simulink model "SatelliteServicing_Mission_RigidBodyTree"  (R2022a)
settings: Solver=ode15s  StartTime=0.0  StopTime=endTime  RelTol=1e-3
libraries: nesl_utility x18, sm_lib x3, robotmaniplib x2
settings Model: Creator=Andy  LastModifiedBy=Andy
settings DebuggingCC: UnconnectedInputMsg=warning  UnconnectedOutputMsg=warning  UnconnectedLineMsg=warning
settings RTWCC: DLArmComputeVersion=19.05
settings SimscapeCC: SimscapeLogType=all

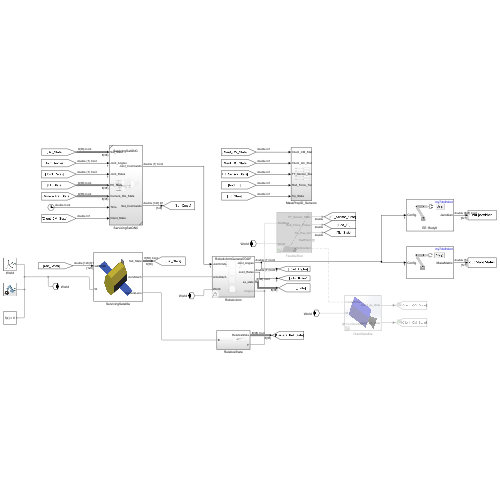
[thumbnail: Simulink's stored preview of the top-level diagram]
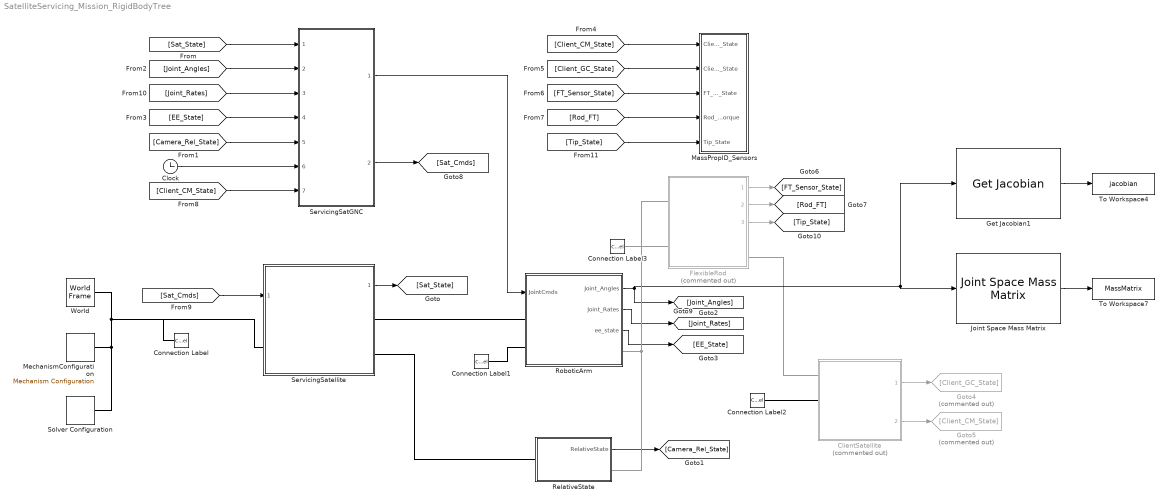
== system SatelliteServicing_Mission_RigidBodyTree ==
  ClientSatellite : Subsystem  Commented=on  ReferencedSubsystem=ClientSatellite
  Clock : Clock
  Connection Label{,1..3} (4 alike) : ConnectionLabel  Label=World
  FlexibleRod : Subsystem  Commented=on  ReferencedSubsystem=FlexibleRodModel
  Get Jacobian1 : robotmaniplib/Get Jacobian  RigidBodyTree=my7dofrobot  EndEffector=Body8  SimulateUsing=Interpreted execution
      settings: SourceProductBaseCode=RO
  Goto4 : Goto  Commented=on  GotoTag=Client_GC_State
  Goto5 : Goto  Commented=on  GotoTag=Client_CM_State
  Joint Space Mass Matrix : robotmaniplib/Joint Space Mass Matrix  RigidBodyTree=my7dofrobot  SimulateUsing=Interpreted execution
  MassPropID_Sensors : Subsystem
  MechanismConfiguration : sm_lib/Utilities/Mechanism Configuration  UniformGravity=Constant  GravityVector=[0 0 -9.80665]*0  GravityUnits=m/s^2  LinearizationDelta=0.001  JointModeTransitionNonlinearIterations=2
  RelativeState : Subsystem
  RoboticArm : Subsystem  Variant=on  VariantControl=Choice
  ServicingSatGNC : Subsystem  SystemSampleTime=0.001  ReferencedSubsystem=ServicingSatGNC
      settings: MinAlgLoopOccurrences=on
  ServicingSatellite : Subsystem  ReferencedSubsystem=ServicingSatellite
  Solver Configuration : nesl_utility/Solver Configuration  PhysicalDomain=network_engine_domain  SubClassName=solver  LeftPortType=input  RightPortType=generic  Tones=[]  Harmonics=[]  SimulateNoise=off  Profile=off  UseLocalSampling=off  EnableSwitchedLinearOptims=on  FrequencyDomain=off  UseCCode=off  RelTol=0.001  AbsTol=1e-06  MinStep=1e-09  ToWorkspace=off  RevertToSquareIcSolve=off  NumHomotopyIterations=100  PhasorMode=off  PhasorModeNumHarmonics=1  IndexReductionMethod=DerivativeReplacement  DoDC=off  ResidualTolerance=1e-09  UseLocalSolver=off  LocalSolverChoice=NE_BACKWARD_EULER_ADVANCER  LocalSolverSampleTime=0.001  DoFixedCost=off  MaxNonlinIter=3  MaxModeIter=2  ComputeImpulses=off  ImpulseIterations=2  LinearAlgebra=auto  LinearAlgebraNumThread=0  EquationFormulation=NE_TIME_EF  DelaysMemoryBudget=1024  AutomaticFiltering=on  FilteringTimeConstant=0.001  PartitionStorageMethod=AS_NEEDED  PartitionMemoryBudget=1024  PartitionMethod=ROBUST
      settings: SourceProductBaseCode=SS,PW,VE
  To Workspace4 : ToWorkspace  VariableName=jacobian  SaveFormat=Timeseries  SampleTime=-1
  To Workspace7 : ToWorkspace  VariableName=MassMatrix  SaveFormat=Timeseries  SampleTime=-1
  World : sm_lib/Frames and Transforms/World Frame
  wires:
  ServicingSatellite/1 -> [Sat_State]
  RelativeState/1(RelativeState) -> [Camera_Rel_State]
  ClientSatellite/1 -> Goto4/1
  FlexibleRod/1 -> [FT_Sensor_State]
  FlexibleRod/2 -> [Rod_FT]
  [Client_CM_State] -> MassPropID_Sensors/1(Client_CM_State)
  [Client_GC_State] -> MassPropID_Sensors/2(Client_GC_State)
  [FT_Sensor_State] -> MassPropID_Sensors/3(FT_Sensor_State)
  [Rod_FT] -> MassPropID_Sensors/4(Rod_Force_Torque)
  [Sat_Cmds] -> ServicingSatellite/1
  ServicingSatGNC/2 -> [Sat_Cmds]
  [Client_CM_State] -> ServicingSatGNC/7
  [Camera_Rel_State] -> ServicingSatGNC/5
  [EE_State] -> ServicingSatGNC/4
  [Sat_State] -> ServicingSatGNC/1
  [Joint_Angles] -> ServicingSatGNC/2
  Clock/1 -> ServicingSatGNC/6
  [Joint_Rates] -> ServicingSatGNC/3
  ServicingSatGNC/1 -> RoboticArm/1(JointCmds)
  RoboticArm/1(Joint_Angles) -> [Joint_Angles], Get Jacobian1/1, Joint Space Mass Matrix/1
  RoboticArm/2(Joint_Rates) -> [Joint_Rates]
  RoboticArm/3(ee_state) -> [EE_State]
  FlexibleRod/3 -> [Tip_State]
  [Tip_State] -> MassPropID_Sensors/5(Tip_State)
  ClientSatellite/2 -> Goto5/1
  Get Jacobian1/1 -> To Workspace4/1
  Joint Space Mass Matrix/1 -> To Workspace7/1
  connections:
  MechanismConfiguration/RConn1 -- ServicingSatellite/LConn1 -- Connection Label/LConn1 -- World/RConn1 -- Solver Configuration/RConn1
  FlexibleRod/RConn2 -- ClientSatellite/LConn1
  RelativeState/LConn1 -- ServicingSatellite/RConn2
  Connection Label2/LConn1 -- ClientSatellite/LConn2
  FlexibleRod/LConn2 -- Connection Label3/LConn1
  RoboticArm/LConn1 -- ServicingSatellite/RConn1
  RoboticArm/LConn2 -- Connection Label1/LConn1
  FlexibleRod/LConn1 -- RelativeState/RConn1 -- RoboticArm/RConn1

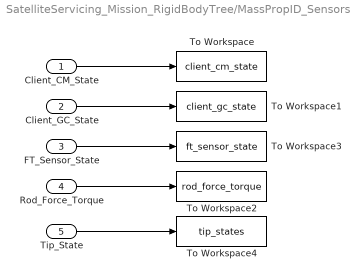
== system SatelliteServicing_Mission_RigidBodyTree/MassPropID_Sensors ==
  Client_CM_State : Inport
  Client_GC_State : Inport  Port=2
  FT_Sensor_State : Inport  Port=3
  Rod_Force_Torque : Inport  Port=4
  Tip_State : Inport  Port=5
  To Workspace : ToWorkspace  VariableName=client_cm_state  SaveFormat=Timeseries  SampleTime=-1
  To Workspace1 : ToWorkspace  VariableName=client_gc_state  SaveFormat=Timeseries  SampleTime=-1
  To Workspace2 : ToWorkspace  VariableName=rod_force_torque  SaveFormat=Timeseries  SampleTime=-1
  To Workspace3 : ToWorkspace  VariableName=ft_sensor_state  SaveFormat=Timeseries  SampleTime=-1
  To Workspace4 : ToWorkspace  VariableName=tip_states  SaveFormat=Timeseries  SampleTime=-1
  wires:
  Rod_Force_Torque/1 -> To Workspace2/1
  Client_CM_State/1 -> To Workspace/1
  Client_GC_State/1 -> To Workspace1/1
  FT_Sensor_State/1 -> To Workspace3/1
  Tip_State/1 -> To Workspace4/1

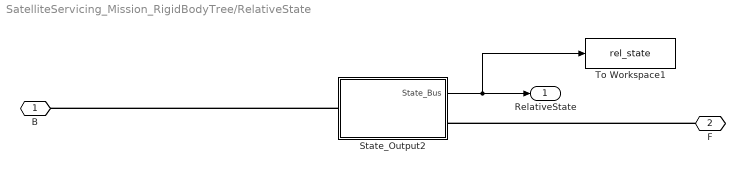
== system SatelliteServicing_Mission_RigidBodyTree/RelativeState ==
  State_Output2 : Subsystem
  To Workspace1 : ToWorkspace  VariableName=rel_state  SaveFormat=Timeseries  SampleTime=-1
  B : PMIOPort  Side=Left
  F : PMIOPort  Port=2  Side=Right
  RelativeState : Outport
  wires:
  State_Output2/1(State_Bus) -> To Workspace1/1, RelativeState/1
  connections:
  F/RConn1 -- State_Output2/RConn1
  State_Output2/LConn1 -- B/RConn1

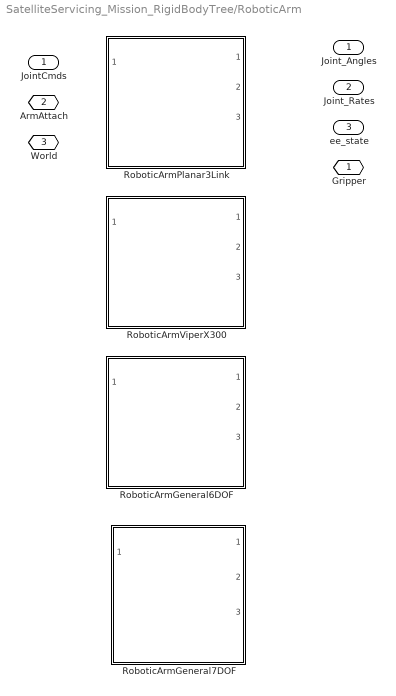
== system SatelliteServicing_Mission_RigidBodyTree/RoboticArm ==
  JointCmds : Inport
  RoboticArmGeneral6DOF : Subsystem  VariantControl=VSS_RoboticArmGeneral6DOF  ReferencedSubsystem=RoboticArmGeneral6DOF
  RoboticArmGeneral7DOF : Subsystem  VariantControl=VSS_RoboticArmGeneral7DOF  ReferencedSubsystem=RoboticArmGeneral7DOF
  RoboticArmPlanar3Link : Subsystem  VariantControl=VSS_RoboticArmPlanar3Link  ReferencedSubsystem=RoboticArmPlanar3Link
  RoboticArmViperX300 : Subsystem  VariantControl=VSS_RoboticArmViperX300  ReferencedSubsystem=RoboticArmViperX300
  Gripper : PMIOPort  Side=Right
  ArmAttach : PMIOPort  Port=2  Side=Left
  World : PMIOPort  Port=3  Side=Left
  Joint_Angles : Outport
  Joint_Rates : Outport  Port=2
  ee_state : Outport  Port=3

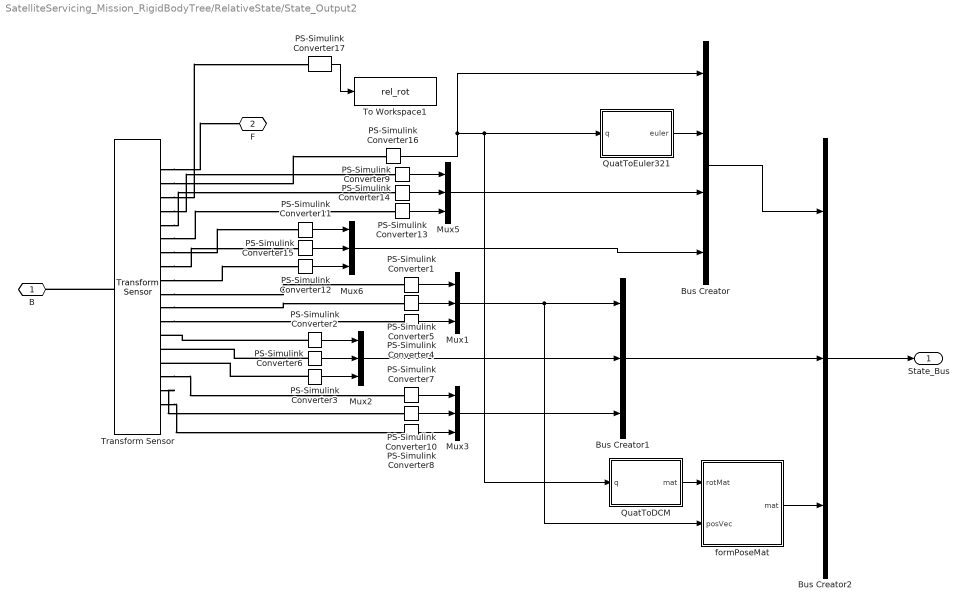
== system SatelliteServicing_Mission_RigidBodyTree/RelativeState/State_Output2 ==
  Bus Creator : BusCreator  Inputs=4  OutDataTypeStr=Bus: RotStateBus
      settings: InheritFromInputs=off
  Bus Creator1 : BusCreator  Inputs=3  OutDataTypeStr=Bus: TransStateBus
      settings: InheritFromInputs=off
  Bus Creator2 : BusCreator  Inputs=3  OutDataTypeStr=Bus: StateBus
      settings: InheritFromInputs=off
  Mux{1..3,5..6} (5 alike) : Mux  Inputs=3
  PS-Simulink Converter{1..17} (17 alike) : nesl_utility/PS-Simulink Converter  PhysicalDomain=network_engine_domain  SubClassName=ps_output  LeftPortType=input  RightPortType=output  PseudoPeriodic=off  Frequencies=[]  VectorFormat=1-D array  Unit=inherit  AffineConversion=off
      settings: SourceProductBaseCode=SS,PW,VE
  QuatToDCM : MATLAB Function  TreatAsAtomicUnit=on
  QuatToEuler321 : MATLAB Function  TreatAsAtomicUnit=on
  To Workspace1 : ToWorkspace  VariableName=rel_rot  SaveFormat=Timeseries  SampleTime=-1
  Transform Sensor : sm_lib/Frames and Transforms/Transform Sensor  MeasurementFrame=Base  SenseAngle=off  SenseAxis=off  SenseAngle1=off  SenseAngle2=off  SenseAngle3=off  SenseQ=on  SenseR=on  SenseOmegaX=on  SenseOmegaY=on  SenseOmegaZ=on  SenseOmega1=off  SenseOmega2=off  SenseOmega3=off  SenseQDot=off  SenseRDot=off  SenseAlphaX=on  SenseAlphaY=on  SenseAlphaZ=on  SenseAlpha1=off  SenseAlpha2=off  SenseAlpha3=off  SenseQDDot=off  SenseRDDot=off  SenseX=on  SenseY=on  SenseZ=on  SenseRad=off  SenseAzim=off  SenseDist=off  SenseInc=off  SenseXDot=on  SenseYDot=on  SenseZDot=on  SenseRadDot=off  SenseAzimDot=off  SenseDistDot=off  SenseIncDot=off  SenseXDDot=on  SenseYDDot=on  SenseZDDot=on  SenseRadDDot=off  SenseAzimDDot=off  SenseDistDDot=off  SenseIncDDot=off
  formPoseMat : MATLAB Function  TreatAsAtomicUnit=on
  B : PMIOPort  Side=Left
  F : PMIOPort  Port=2  Side=Right
  State_Bus : Outport
  wires:
  PS-Simulink Converter4/1 -> Mux1/3
  PS-Simulink Converter5/1 -> Mux1/2
  PS-Simulink Converter1/1 -> Mux1/1
  PS-Simulink Converter3/1 -> Mux2/3
  PS-Simulink Converter6/1 -> Mux2/2
  PS-Simulink Converter2/1 -> Mux2/1
  PS-Simulink Converter10/1 -> Mux3/2
  PS-Simulink Converter8/1 -> Mux3/3
  PS-Simulink Converter7/1 -> Mux3/1
  Mux2/1 -> Bus Creator1/2
  Mux1/1 -> formPoseMat/2(posVec), Bus Creator1/1
  Mux3/1 -> Bus Creator1/3
  PS-Simulink Converter9/1 -> Mux5/1
  PS-Simulink Converter14/1 -> Mux5/2
  PS-Simulink Converter13/1 -> Mux5/3
  Mux5/1 -> Bus Creator/3
  PS-Simulink Converter15/1 -> Mux6/2
  PS-Simulink Converter12/1 -> Mux6/3
  Mux6/1 -> Bus Creator/4
  PS-Simulink Converter11/1 -> Mux6/1
  PS-Simulink Converter16/1 -> QuatToEuler321/1(q), QuatToDCM/1(q), Bus Creator/1
  QuatToEuler321/1(euler) -> Bus Creator/2
  Bus Creator/1 -> Bus Creator2/1
  Bus Creator1/1 -> Bus Creator2/2
  Bus Creator2/1 -> State_Bus/1
  QuatToDCM/1(mat) -> formPoseMat/1(rotMat)
  formPoseMat/1(mat) -> Bus Creator2/3
  PS-Simulink Converter17/1 -> To Workspace1/1
  connections:
  Transform Sensor/LConn1 -- B/RConn1
  Transform Sensor/RConn1 -- F/RConn1
  Transform Sensor/RConn10 -- PS-Simulink Converter1/LConn1
  Transform Sensor/RConn11 -- PS-Simulink Converter5/LConn1
  Transform Sensor/RConn12 -- PS-Simulink Converter4/LConn1
  PS-Simulink Converter3/LConn1 -- Transform Sensor/RConn15
  PS-Simulink Converter6/LConn1 -- Transform Sensor/RConn14
  PS-Simulink Converter2/LConn1 -- Transform Sensor/RConn13
  Transform Sensor/RConn18 -- PS-Simulink Converter8/LConn1
  Transform Sensor/RConn16 -- PS-Simulink Converter7/LConn1
  Transform Sensor/RConn17 -- PS-Simulink Converter10/LConn1
  Transform Sensor/RConn9 -- PS-Simulink Converter12/LConn1
  Transform Sensor/RConn6 -- PS-Simulink Converter13/LConn1
  Transform Sensor/RConn5 -- PS-Simulink Converter14/LConn1
  Transform Sensor/RConn4 -- PS-Simulink Converter9/LConn1
  Transform Sensor/RConn8 -- PS-Simulink Converter15/LConn1
  Transform Sensor/RConn7 -- PS-Simulink Converter11/LConn1
  Transform Sensor/RConn2 -- PS-Simulink Converter16/LConn1
  Transform Sensor/RConn3 -- PS-Simulink Converter17/LConn1

== matlab function SatelliteServicing_Mission_RigidBodyTree/RelativeState/State_Output2/QuatToDCM ==
  data: q input; mat output
function mat  = callQuatToDCM(q)

[mat] = simscapeQuatToDCM(q);

== matlab function SatelliteServicing_Mission_RigidBodyTree/RelativeState/State_Output2/QuatToEuler321 ==
  data: q input; euler output
function euler  = callQuatToEuler321(q)


[euler] = quatToEuler_321(q);

== matlab function SatelliteServicing_Mission_RigidBodyTree/RelativeState/State_Output2/formPoseMat ==
  data: rotMat input; mat output; posVec input
function mat  = callFormPoseMat(rotMat,posVec)


[mat] = formPoseMat(rotMat,posVec);
